simulink model "Byte_Demultiplexers"  (Simulink 8.1)
settings: Solver=ode45  StartTime=0.0  StopTime=10.0  RelTol=1e-3
libraries: Common_Library x32, commutil2 x22, Computer_Library x17
settings Model: Creator=uzivatel  LastModifiedBy=uzivatel
settings DataIOCC: SignalLoggingSaveFormat=Dataset
settings OptimizationCC: ExpressionDepthLimit=128
settings DebuggingCC: FcnCallInpInsideContextMsg=EnableAllAsError
settings GRTTargetCC: CombineOutputUpdateFcns=on  GRTInterface=off

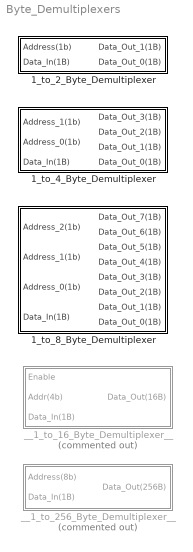
== system Byte_Demultiplexers ==
  1_to_2_Byte_Demultiplexer : Subsystem
  1_to_4_Byte_Demultiplexer : Subsystem
  1_to_8_Byte_Demultiplexer : Subsystem
  __1_to_16_Byte_Demultiplexer__ : Subsystem  Commented=on
  __1_to_256_Byte_Demultiplexer__ : Subsystem  Commented=on

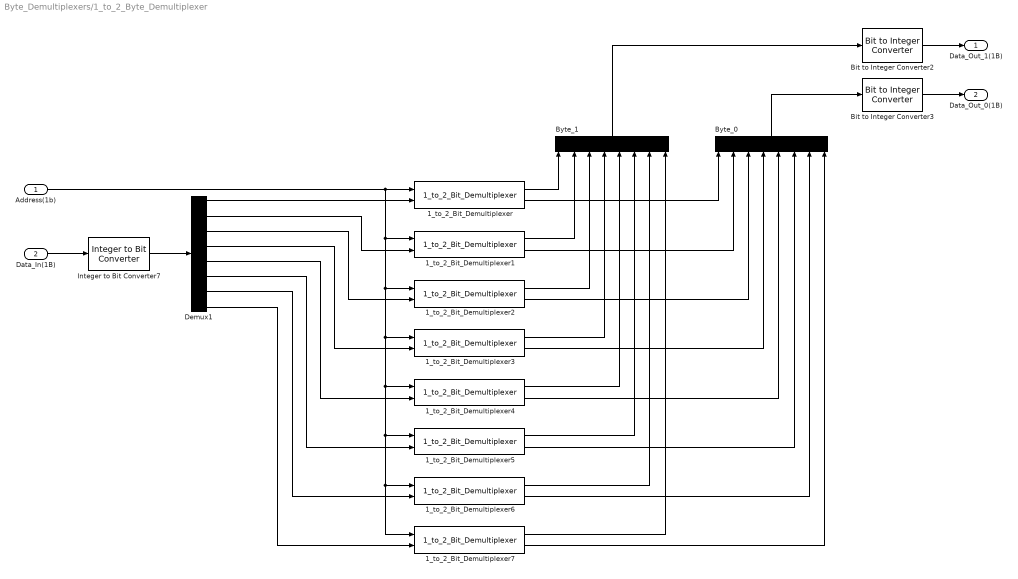
== system Byte_Demultiplexers/1_to_2_Byte_Demultiplexer ==
  Address(1b) : Inport
  Data_In(1B) : Inport  Port=2
  1_to_2_Bit_Demultiplexer{,1..7} (8 alike) : Common_Library/Demultiplexers/1_to_2_Bit_Demultiplexer
  Bit to Integer Converter2 : commutil2/Bit to Integer Converter  nbits=8  bitOrder=MSB first  signedOutputValues=Unsigned  outDtype=uint8  outDtypeSigned=Inherit via internal rule
  Bit to Integer Converter3 : commutil2/Bit to Integer Converter  nbits=8  bitOrder=MSB first  signedOutputValues=Unsigned  outDtype=uint8  outDtypeSigned=Inherit via internal rule
  Byte_0 : Mux  Inputs=8
  Byte_1 : Mux  Inputs=8
  Demux1 : Demux  Outputs=8
  Integer to Bit Converter7 : commutil2/Integer to Bit Converter  nbits=8  signedInputValues=Unsigned  bitOrder=MSB first  outDtype=boolean
  Data_Out_1(1B) : Outport
  Data_Out_0(1B) : Outport  Port=2
  wires:
  Demux1/4 -> 1_to_2_Bit_Demultiplexer3/2
  Demux1/5 -> 1_to_2_Bit_Demultiplexer4/2
  Demux1/6 -> 1_to_2_Bit_Demultiplexer5/2
  Demux1/7 -> 1_to_2_Bit_Demultiplexer6/2
  Demux1/8 -> 1_to_2_Bit_Demultiplexer7/2
  Demux1/3 -> 1_to_2_Bit_Demultiplexer2/2
  Demux1/2 -> 1_to_2_Bit_Demultiplexer1/2
  Demux1/1 -> 1_to_2_Bit_Demultiplexer/2
  Byte_1/1 -> Bit to Integer Converter2/1
  Byte_0/1 -> Bit to Integer Converter3/1
  1_to_2_Bit_Demultiplexer7/2 -> Byte_0/8
  1_to_2_Bit_Demultiplexer7/1 -> Byte_1/8
  1_to_2_Bit_Demultiplexer6/2 -> Byte_0/7
  1_to_2_Bit_Demultiplexer6/1 -> Byte_1/7
  1_to_2_Bit_Demultiplexer5/2 -> Byte_0/6
  1_to_2_Bit_Demultiplexer5/1 -> Byte_1/6
  1_to_2_Bit_Demultiplexer4/2 -> Byte_0/5
  1_to_2_Bit_Demultiplexer4/1 -> Byte_1/5
  1_to_2_Bit_Demultiplexer3/2 -> Byte_0/4
  1_to_2_Bit_Demultiplexer3/1 -> Byte_1/4
  1_to_2_Bit_Demultiplexer2/2 -> Byte_0/3
  1_to_2_Bit_Demultiplexer2/1 -> Byte_1/3
  1_to_2_Bit_Demultiplexer1/2 -> Byte_0/2
  1_to_2_Bit_Demultiplexer1/1 -> Byte_1/2
  1_to_2_Bit_Demultiplexer/2 -> Byte_0/1
  1_to_2_Bit_Demultiplexer/1 -> Byte_1/1
  Integer to Bit Converter7/1 -> Demux1/1
  Data_In(1B)/1 -> Integer to Bit Converter7/1
  Address(1b)/1 -> 1_to_2_Bit_Demultiplexer/1, 1_to_2_Bit_Demultiplexer7/1, 1_to_2_Bit_Demultiplexer6/1, 1_to_2_Bit_Demultiplexer5/1, 1_to_2_Bit_Demultiplexer4/1, 1_to_2_Bit_Demultiplexer3/1, 1_to_2_Bit_Demultiplexer2/1, 1_to_2_Bit_Demultiplexer1/1
  Bit to Integer Converter2/1 -> Data_Out_1(1B)/1
  Bit to Integer Converter3/1 -> Data_Out_0(1B)/1

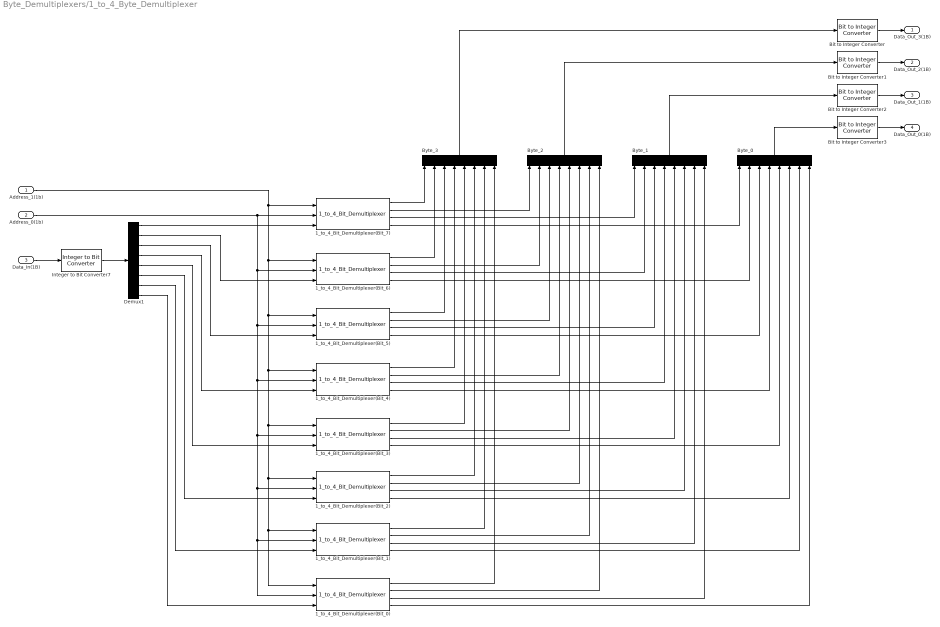
== system Byte_Demultiplexers/1_to_4_Byte_Demultiplexer ==
  Address_1(1b) : Inport
  Address_0(1b) : Inport  Port=2
  Data_In(1B) : Inport  Port=3
  1_to_4_Bit_Demultiplexer(Bit_0) : Common_Library/Demultiplexers/1_to_4_Bit_Demultiplexer
  1_to_4_Bit_Demultiplexer(Bit_1) : Common_Library/Demultiplexers/1_to_4_Bit_Demultiplexer
  1_to_4_Bit_Demultiplexer(Bit_2) : Common_Library/Demultiplexers/1_to_4_Bit_Demultiplexer
  1_to_4_Bit_Demultiplexer(Bit_3) : Common_Library/Demultiplexers/1_to_4_Bit_Demultiplexer
  1_to_4_Bit_Demultiplexer(Bit_4) : Common_Library/Demultiplexers/1_to_4_Bit_Demultiplexer
  1_to_4_Bit_Demultiplexer(Bit_5) : Common_Library/Demultiplexers/1_to_4_Bit_Demultiplexer
  1_to_4_Bit_Demultiplexer(Bit_6) : Common_Library/Demultiplexers/1_to_4_Bit_Demultiplexer
  1_to_4_Bit_Demultiplexer(Bit_7) : Common_Library/Demultiplexers/1_to_4_Bit_Demultiplexer
  Bit to Integer Converter{,1..3} (4 alike) : commutil2/Bit to Integer Converter  nbits=8  bitOrder=MSB first  signedOutputValues=Unsigned  outDtype=uint8  outDtypeSigned=Inherit via internal rule
  Byte_{0..3} (4 alike) : Mux  Inputs=8
  Demux1 : Demux  Outputs=8
  Integer to Bit Converter7 : commutil2/Integer to Bit Converter  nbits=8  signedInputValues=Unsigned  bitOrder=MSB first  outDtype=boolean
  Data_Out_3(1B) : Outport
  Data_Out_2(1B) : Outport  Port=2
  Data_Out_1(1B) : Outport  Port=3
  Data_Out_0(1B) : Outport  Port=4
  wires:
  Bit to Integer Converter/1 -> Data_Out_3(1B)/1
  Demux1/4 -> 1_to_4_Bit_Demultiplexer(Bit_4)/3
  Demux1/5 -> 1_to_4_Bit_Demultiplexer(Bit_3)/3
  Demux1/6 -> 1_to_4_Bit_Demultiplexer(Bit_2)/3
  Demux1/7 -> 1_to_4_Bit_Demultiplexer(Bit_1)/3
  Demux1/8 -> 1_to_4_Bit_Demultiplexer(Bit_0)/3
  Demux1/3 -> 1_to_4_Bit_Demultiplexer(Bit_5)/3
  Demux1/2 -> 1_to_4_Bit_Demultiplexer(Bit_6)/3
  Demux1/1 -> 1_to_4_Bit_Demultiplexer(Bit_7)/3
  Byte_3/1 -> Bit to Integer Converter/1
  Byte_2/1 -> Bit to Integer Converter1/1
  Byte_1/1 -> Bit to Integer Converter2/1
  Byte_0/1 -> Bit to Integer Converter3/1
  1_to_4_Bit_Demultiplexer(Bit_0)/4 -> Byte_0/8
  1_to_4_Bit_Demultiplexer(Bit_0)/3 -> Byte_1/8
  1_to_4_Bit_Demultiplexer(Bit_0)/2 -> Byte_2/8
  1_to_4_Bit_Demultiplexer(Bit_0)/1 -> Byte_3/8
  1_to_4_Bit_Demultiplexer(Bit_1)/4 -> Byte_0/7
  1_to_4_Bit_Demultiplexer(Bit_1)/3 -> Byte_1/7
  1_to_4_Bit_Demultiplexer(Bit_1)/2 -> Byte_2/7
  1_to_4_Bit_Demultiplexer(Bit_1)/1 -> Byte_3/7
  1_to_4_Bit_Demultiplexer(Bit_2)/4 -> Byte_0/6
  1_to_4_Bit_Demultiplexer(Bit_2)/3 -> Byte_1/6
  1_to_4_Bit_Demultiplexer(Bit_2)/2 -> Byte_2/6
  1_to_4_Bit_Demultiplexer(Bit_2)/1 -> Byte_3/6
  1_to_4_Bit_Demultiplexer(Bit_3)/4 -> Byte_0/5
  1_to_4_Bit_Demultiplexer(Bit_3)/3 -> Byte_1/5
  1_to_4_Bit_Demultiplexer(Bit_3)/2 -> Byte_2/5
  1_to_4_Bit_Demultiplexer(Bit_3)/1 -> Byte_3/5
  1_to_4_Bit_Demultiplexer(Bit_4)/4 -> Byte_0/4
  1_to_4_Bit_Demultiplexer(Bit_4)/3 -> Byte_1/4
  1_to_4_Bit_Demultiplexer(Bit_4)/2 -> Byte_2/4
  1_to_4_Bit_Demultiplexer(Bit_4)/1 -> Byte_3/4
  1_to_4_Bit_Demultiplexer(Bit_5)/4 -> Byte_0/3
  1_to_4_Bit_Demultiplexer(Bit_5)/3 -> Byte_1/3
  1_to_4_Bit_Demultiplexer(Bit_5)/2 -> Byte_2/3
  1_to_4_Bit_Demultiplexer(Bit_5)/1 -> Byte_3/3
  1_to_4_Bit_Demultiplexer(Bit_6)/4 -> Byte_0/2
  1_to_4_Bit_Demultiplexer(Bit_6)/3 -> Byte_1/2
  1_to_4_Bit_Demultiplexer(Bit_6)/2 -> Byte_2/2
  1_to_4_Bit_Demultiplexer(Bit_6)/1 -> Byte_3/2
  1_to_4_Bit_Demultiplexer(Bit_7)/4 -> Byte_0/1
  1_to_4_Bit_Demultiplexer(Bit_7)/3 -> Byte_1/1
  1_to_4_Bit_Demultiplexer(Bit_7)/2 -> Byte_2/1
  1_to_4_Bit_Demultiplexer(Bit_7)/1 -> Byte_3/1
  Integer to Bit Converter7/1 -> Demux1/1
  Data_In(1B)/1 -> Integer to Bit Converter7/1
  Address_0(1b)/1 -> 1_to_4_Bit_Demultiplexer(Bit_7)/2, 1_to_4_Bit_Demultiplexer(Bit_3)/2, 1_to_4_Bit_Demultiplexer(Bit_2)/2, 1_to_4_Bit_Demultiplexer(Bit_1)/2, 1_to_4_Bit_Demultiplexer(Bit_0)/2, 1_to_4_Bit_Demultiplexer(Bit_4)/2, 1_to_4_Bit_Demultiplexer(Bit_5)/2, 1_to_4_Bit_Demultiplexer(Bit_6)/2
  Address_1(1b)/1 -> 1_to_4_Bit_Demultiplexer(Bit_7)/1, 1_to_4_Bit_Demultiplexer(Bit_0)/1, 1_to_4_Bit_Demultiplexer(Bit_1)/1, 1_to_4_Bit_Demultiplexer(Bit_2)/1, 1_to_4_Bit_Demultiplexer(Bit_3)/1, 1_to_4_Bit_Demultiplexer(Bit_4)/1, 1_to_4_Bit_Demultiplexer(Bit_5)/1, 1_to_4_Bit_Demultiplexer(Bit_6)/1
  Bit to Integer Converter1/1 -> Data_Out_2(1B)/1
  Bit to Integer Converter2/1 -> Data_Out_1(1B)/1
  Bit to Integer Converter3/1 -> Data_Out_0(1B)/1

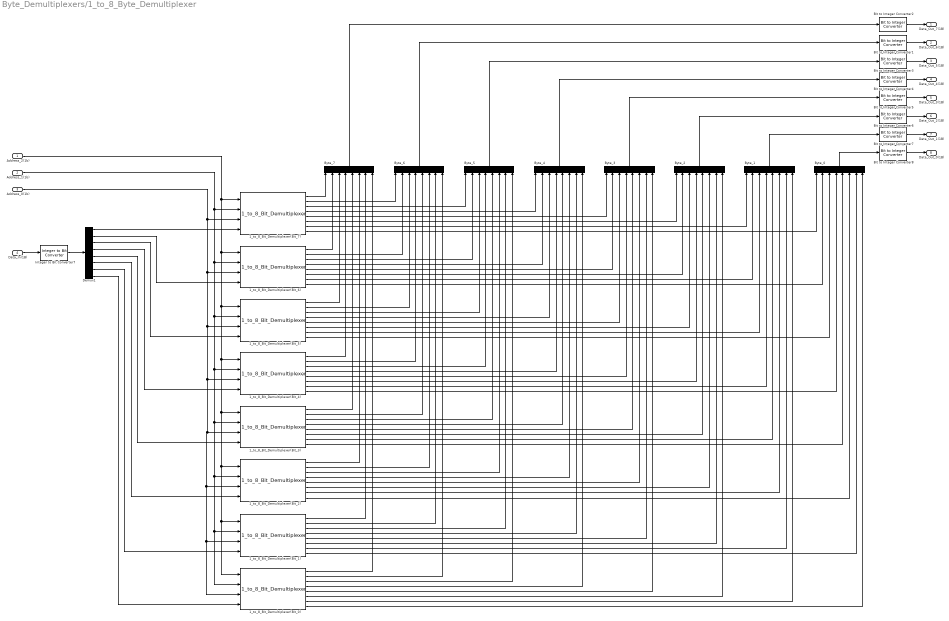
== system Byte_Demultiplexers/1_to_8_Byte_Demultiplexer ==
  Address_2(1b) : Inport
  Address_1(1b) : Inport  Port=2
  Address_0(1b) : Inport  Port=3
  Data_In(1B) : Inport  Port=4
  1_to_8_Bit_Demultiplexer(Bit_0) : Common_Library/Demultiplexers/1_to_8_Bit_Demultiplexer
  1_to_8_Bit_Demultiplexer(Bit_1) : Common_Library/Demultiplexers/1_to_8_Bit_Demultiplexer
  1_to_8_Bit_Demultiplexer(Bit_2) : Common_Library/Demultiplexers/1_to_8_Bit_Demultiplexer
  1_to_8_Bit_Demultiplexer(Bit_3) : Common_Library/Demultiplexers/1_to_8_Bit_Demultiplexer
  1_to_8_Bit_Demultiplexer(Bit_4) : Common_Library/Demultiplexers/1_to_8_Bit_Demultiplexer
  1_to_8_Bit_Demultiplexer(Bit_5) : Common_Library/Demultiplexers/1_to_8_Bit_Demultiplexer
  1_to_8_Bit_Demultiplexer(Bit_6) : Common_Library/Demultiplexers/1_to_8_Bit_Demultiplexer
  1_to_8_Bit_Demultiplexer(Bit_7) : Common_Library/Demultiplexers/1_to_8_Bit_Demultiplexer
  Bit to Integer Converter{1..8} (8 alike) : commutil2/Bit to Integer Converter  nbits=8  bitOrder=MSB first  signedOutputValues=Unsigned  outDtype=uint8  outDtypeSigned=Inherit via internal rule
  Byte_{0..7} (8 alike) : Mux  Inputs=8
  Demux1 : Demux  Outputs=8
  Integer to Bit Converter7 : commutil2/Integer to Bit Converter  nbits=8  signedInputValues=Unsigned  bitOrder=MSB first  outDtype=boolean
  Data_Out_7(1B) : Outport
  Data_Out_6(1B) : Outport  Port=2
  Data_Out_5(1B) : Outport  Port=3
  Data_Out_4(1B) : Outport  Port=4
  Data_Out_3(1B) : Outport  Port=5
  Data_Out_2(1B) : Outport  Port=6
  Data_Out_1(1B) : Outport  Port=7
  Data_Out_0(1B) : Outport  Port=8
  wires:
  Demux1/4 -> 1_to_8_Bit_Demultiplexer(Bit_4)/4
  Demux1/5 -> 1_to_8_Bit_Demultiplexer(Bit_3)/4
  Demux1/6 -> 1_to_8_Bit_Demultiplexer(Bit_2)/4
  Demux1/7 -> 1_to_8_Bit_Demultiplexer(Bit_1)/4
  Demux1/8 -> 1_to_8_Bit_Demultiplexer(Bit_0)/4
  Demux1/3 -> 1_to_8_Bit_Demultiplexer(Bit_5)/4
  Demux1/2 -> 1_to_8_Bit_Demultiplexer(Bit_6)/4
  Demux1/1 -> 1_to_8_Bit_Demultiplexer(Bit_7)/4
  Byte_7/1 -> Bit to Integer Converter2/1
  Byte_6/1 -> Bit to Integer Converter1/1
  Byte_5/1 -> Bit to Integer Converter3/1
  Byte_4/1 -> Bit to Integer Converter4/1
  Byte_3/1 -> Bit to Integer Converter5/1
  Byte_2/1 -> Bit to Integer Converter6/1
  Byte_1/1 -> Bit to Integer Converter7/1
  Byte_0/1 -> Bit to Integer Converter8/1
  1_to_8_Bit_Demultiplexer(Bit_0)/8 -> Byte_0/8
  1_to_8_Bit_Demultiplexer(Bit_0)/7 -> Byte_1/8
  1_to_8_Bit_Demultiplexer(Bit_0)/6 -> Byte_2/8
  1_to_8_Bit_Demultiplexer(Bit_0)/5 -> Byte_3/8
  1_to_8_Bit_Demultiplexer(Bit_0)/4 -> Byte_4/8
  1_to_8_Bit_Demultiplexer(Bit_0)/3 -> Byte_5/8
  1_to_8_Bit_Demultiplexer(Bit_0)/2 -> Byte_6/8
  1_to_8_Bit_Demultiplexer(Bit_0)/1 -> Byte_7/8
  1_to_8_Bit_Demultiplexer(Bit_1)/8 -> Byte_0/7
  1_to_8_Bit_Demultiplexer(Bit_1)/7 -> Byte_1/7
  1_to_8_Bit_Demultiplexer(Bit_1)/6 -> Byte_2/7
  1_to_8_Bit_Demultiplexer(Bit_1)/5 -> Byte_3/7
  1_to_8_Bit_Demultiplexer(Bit_1)/4 -> Byte_4/7
  1_to_8_Bit_Demultiplexer(Bit_1)/3 -> Byte_5/7
  1_to_8_Bit_Demultiplexer(Bit_1)/2 -> Byte_6/7
  1_to_8_Bit_Demultiplexer(Bit_1)/1 -> Byte_7/7
  1_to_8_Bit_Demultiplexer(Bit_2)/8 -> Byte_0/6
  1_to_8_Bit_Demultiplexer(Bit_2)/7 -> Byte_1/6
  1_to_8_Bit_Demultiplexer(Bit_2)/6 -> Byte_2/6
  1_to_8_Bit_Demultiplexer(Bit_2)/5 -> Byte_3/6
  1_to_8_Bit_Demultiplexer(Bit_2)/4 -> Byte_4/6
  1_to_8_Bit_Demultiplexer(Bit_2)/3 -> Byte_5/6
  1_to_8_Bit_Demultiplexer(Bit_2)/2 -> Byte_6/6
  1_to_8_Bit_Demultiplexer(Bit_2)/1 -> Byte_7/6
  1_to_8_Bit_Demultiplexer(Bit_3)/8 -> Byte_0/5
  1_to_8_Bit_Demultiplexer(Bit_3)/7 -> Byte_1/5
  1_to_8_Bit_Demultiplexer(Bit_3)/6 -> Byte_2/5
  1_to_8_Bit_Demultiplexer(Bit_3)/5 -> Byte_3/5
  1_to_8_Bit_Demultiplexer(Bit_3)/4 -> Byte_4/5
  1_to_8_Bit_Demultiplexer(Bit_3)/3 -> Byte_5/5
  1_to_8_Bit_Demultiplexer(Bit_3)/2 -> Byte_6/5
  1_to_8_Bit_Demultiplexer(Bit_3)/1 -> Byte_7/5
  1_to_8_Bit_Demultiplexer(Bit_4)/8 -> Byte_0/4
  1_to_8_Bit_Demultiplexer(Bit_4)/7 -> Byte_1/4
  1_to_8_Bit_Demultiplexer(Bit_4)/6 -> Byte_2/4
  1_to_8_Bit_Demultiplexer(Bit_4)/5 -> Byte_3/4
  1_to_8_Bit_Demultiplexer(Bit_4)/4 -> Byte_4/4
  1_to_8_Bit_Demultiplexer(Bit_4)/3 -> Byte_5/4
  1_to_8_Bit_Demultiplexer(Bit_4)/2 -> Byte_6/4
  1_to_8_Bit_Demultiplexer(Bit_4)/1 -> Byte_7/4
  1_to_8_Bit_Demultiplexer(Bit_5)/8 -> Byte_0/3
  1_to_8_Bit_Demultiplexer(Bit_5)/7 -> Byte_1/3
  1_to_8_Bit_Demultiplexer(Bit_5)/6 -> Byte_2/3
  1_to_8_Bit_Demultiplexer(Bit_5)/5 -> Byte_3/3
  1_to_8_Bit_Demultiplexer(Bit_5)/4 -> Byte_4/3
  1_to_8_Bit_Demultiplexer(Bit_5)/3 -> Byte_5/3
  1_to_8_Bit_Demultiplexer(Bit_5)/2 -> Byte_6/3
  1_to_8_Bit_Demultiplexer(Bit_5)/1 -> Byte_7/3
  1_to_8_Bit_Demultiplexer(Bit_6)/8 -> Byte_0/2
  1_to_8_Bit_Demultiplexer(Bit_6)/7 -> Byte_1/2
  1_to_8_Bit_Demultiplexer(Bit_6)/6 -> Byte_2/2
  1_to_8_Bit_Demultiplexer(Bit_6)/5 -> Byte_3/2
  1_to_8_Bit_Demultiplexer(Bit_6)/4 -> Byte_4/2
  1_to_8_Bit_Demultiplexer(Bit_6)/3 -> Byte_5/2
  1_to_8_Bit_Demultiplexer(Bit_6)/2 -> Byte_6/2
  1_to_8_Bit_Demultiplexer(Bit_6)/1 -> Byte_7/2
  1_to_8_Bit_Demultiplexer(Bit_7)/8 -> Byte_0/1
  1_to_8_Bit_Demultiplexer(Bit_7)/7 -> Byte_1/1
  1_to_8_Bit_Demultiplexer(Bit_7)/6 -> Byte_2/1
  1_to_8_Bit_Demultiplexer(Bit_7)/5 -> Byte_3/1
  1_to_8_Bit_Demultiplexer(Bit_7)/4 -> Byte_4/1
  1_to_8_Bit_Demultiplexer(Bit_7)/3 -> Byte_5/1
  1_to_8_Bit_Demultiplexer(Bit_7)/2 -> Byte_6/1
  1_to_8_Bit_Demultiplexer(Bit_7)/1 -> Byte_7/1
  Integer to Bit Converter7/1 -> Demux1/1
  Data_In(1B)/1 -> Integer to Bit Converter7/1
  Address_0(1b)/1 -> 1_to_8_Bit_Demultiplexer(Bit_7)/3, 1_to_8_Bit_Demultiplexer(Bit_6)/3, 1_to_8_Bit_Demultiplexer(Bit_5)/3, 1_to_8_Bit_Demultiplexer(Bit_0)/3, 1_to_8_Bit_Demultiplexer(Bit_1)/3, 1_to_8_Bit_Demultiplexer(Bit_2)/3, 1_to_8_Bit_Demultiplexer(Bit_3)/3, 1_to_8_Bit_Demultiplexer(Bit_4)/3
  Address_1(1b)/1 -> 1_to_8_Bit_Demultiplexer(Bit_7)/2, 1_to_8_Bit_Demultiplexer(Bit_0)/2, 1_to_8_Bit_Demultiplexer(Bit_1)/2, 1_to_8_Bit_Demultiplexer(Bit_2)/2, 1_to_8_Bit_Demultiplexer(Bit_3)/2, 1_to_8_Bit_Demultiplexer(Bit_4)/2, 1_to_8_Bit_Demultiplexer(Bit_5)/2, 1_to_8_Bit_Demultiplexer(Bit_6)/2
  Address_2(1b)/1 -> 1_to_8_Bit_Demultiplexer(Bit_7)/1, 1_to_8_Bit_Demultiplexer(Bit_0)/1, 1_to_8_Bit_Demultiplexer(Bit_1)/1, 1_to_8_Bit_Demultiplexer(Bit_2)/1, 1_to_8_Bit_Demultiplexer(Bit_3)/1, 1_to_8_Bit_Demultiplexer(Bit_4)/1, 1_to_8_Bit_Demultiplexer(Bit_5)/1, 1_to_8_Bit_Demultiplexer(Bit_6)/1
  Bit to Integer Converter8/1 -> Data_Out_0(1B)/1
  Bit to Integer Converter7/1 -> Data_Out_1(1B)/1
  Bit to Integer Converter6/1 -> Data_Out_2(1B)/1
  Bit to Integer Converter5/1 -> Data_Out_3(1B)/1
  Bit to Integer Converter4/1 -> Data_Out_4(1B)/1
  Bit to Integer Converter3/1 -> Data_Out_5(1B)/1
  Bit to Integer Converter1/1 -> Data_Out_6(1B)/1
  Bit to Integer Converter2/1 -> Data_Out_7(1B)/1

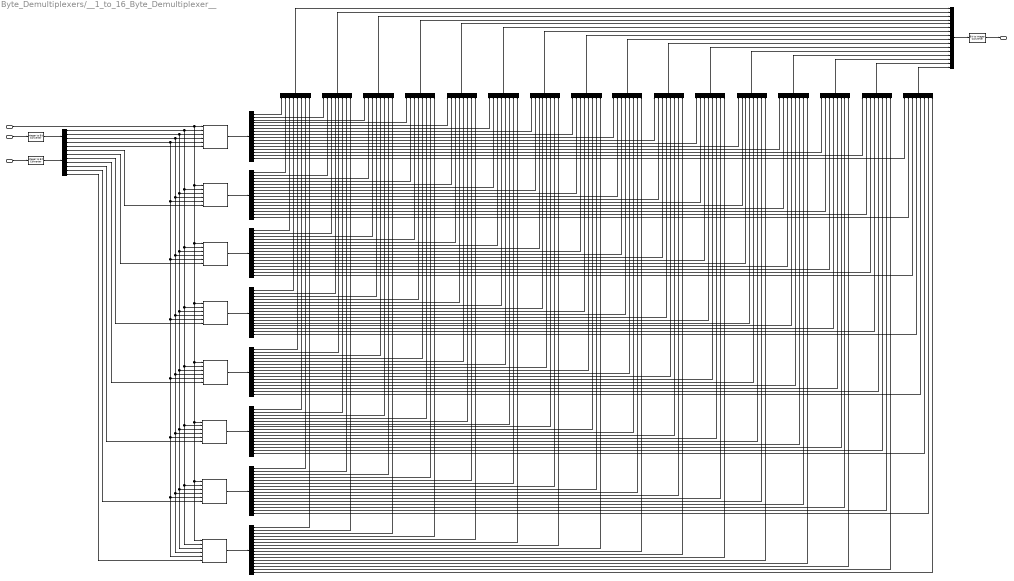
== system Byte_Demultiplexers/__1_to_16_Byte_Demultiplexer__ ==
  Enable : Inport
  Addr(4b) : Inport  Port=2
  Data_In(1B) : Inport  Port=3
  1_to_16_Bit_Demultiplexer(Bit_0) : Common_Library/Demultiplexers/1_to_16_Bit_Demultiplexer
  1_to_16_Bit_Demultiplexer(Bit_1) : Common_Library/Demultiplexers/1_to_16_Bit_Demultiplexer
  1_to_16_Bit_Demultiplexer(Bit_2) : Common_Library/Demultiplexers/1_to_16_Bit_Demultiplexer
  1_to_16_Bit_Demultiplexer(Bit_3) : Common_Library/Demultiplexers/1_to_16_Bit_Demultiplexer
  1_to_16_Bit_Demultiplexer(Bit_4) : Common_Library/Demultiplexers/1_to_16_Bit_Demultiplexer
  1_to_16_Bit_Demultiplexer(Bit_5) : Common_Library/Demultiplexers/1_to_16_Bit_Demultiplexer
  1_to_16_Bit_Demultiplexer(Bit_6) : Common_Library/Demultiplexers/1_to_16_Bit_Demultiplexer
  1_to_16_Bit_Demultiplexer(Bit_7) : Common_Library/Demultiplexers/1_to_16_Bit_Demultiplexer
  Bit to Integer Converter : commutil2/Bit to Integer Converter  nbits=8  bitOrder=MSB first  signedOutputValues=Unsigned  outDtype=uint8  outDtypeSigned=Inherit via internal rule
  Bit_{0..7} (8 alike) : Demux  Outputs=16
  Byte_{0..15} (16 alike) : Mux  Inputs=8
  Demux1 : Demux  Outputs=8
  Demux17 : Demux
  Integer to Bit Converter5 : commutil2/Integer to Bit Converter  nbits=4  signedInputValues=Unsigned  bitOrder=MSB first  outDtype=int8
  Integer to Bit Converter7 : commutil2/Integer to Bit Converter  nbits=8  signedInputValues=Unsigned  bitOrder=MSB first  outDtype=boolean
  Mux1 : Mux  Inputs=16
  Data_Out(16B) : Outport
  wires:
  Bit to Integer Converter/1 -> Data_Out(16B)/1
  Mux1/1 -> Bit to Integer Converter/1
  Addr(4b)/1 -> Integer to Bit Converter5/1
  Integer to Bit Converter5/1 -> Demux17/1
  Enable/1 -> 1_to_16_Bit_Demultiplexer(Bit_0)/1, 1_to_16_Bit_Demultiplexer(Bit_1)/1, 1_to_16_Bit_Demultiplexer(Bit_2)/1, 1_to_16_Bit_Demultiplexer(Bit_3)/1, 1_to_16_Bit_Demultiplexer(Bit_4)/1, 1_to_16_Bit_Demultiplexer(Bit_5)/1, 1_to_16_Bit_Demultiplexer(Bit_6)/1, 1_to_16_Bit_Demultiplexer(Bit_7)/1
  Demux1/4 -> 1_to_16_Bit_Demultiplexer(Bit_4)/6
  Demux1/5 -> 1_to_16_Bit_Demultiplexer(Bit_3)/6
  Demux1/6 -> 1_to_16_Bit_Demultiplexer(Bit_2)/6
  Demux1/7 -> 1_to_16_Bit_Demultiplexer(Bit_1)/6
  Demux1/8 -> 1_to_16_Bit_Demultiplexer(Bit_0)/6
  Demux1/3 -> 1_to_16_Bit_Demultiplexer(Bit_5)/6
  Demux1/2 -> 1_to_16_Bit_Demultiplexer(Bit_6)/6
  Demux1/1 -> 1_to_16_Bit_Demultiplexer(Bit_7)/6
  Byte_15/1 -> Mux1/1
  Byte_14/1 -> Mux1/2
  Byte_13/1 -> Mux1/3
  Byte_12/1 -> Mux1/4
  Byte_11/1 -> Mux1/5
  Byte_10/1 -> Mux1/6
  Byte_9/1 -> Mux1/7
  Byte_8/1 -> Mux1/8
  Byte_7/1 -> Mux1/9
  Byte_6/1 -> Mux1/10
  Byte_5/1 -> Mux1/11
  Byte_4/1 -> Mux1/12
  Byte_3/1 -> Mux1/13
  Byte_2/1 -> Mux1/14
  Byte_1/1 -> Mux1/15
  Byte_0/1 -> Mux1/16
  Bit_0/16 -> Byte_0/8
  Bit_0/15 -> Byte_1/8
  Bit_0/14 -> Byte_2/8
  Bit_0/13 -> Byte_3/8
  Bit_0/12 -> Byte_4/8
  Bit_0/11 -> Byte_5/8
  Bit_0/10 -> Byte_6/8
  Bit_0/9 -> Byte_7/8
  Bit_0/8 -> Byte_8/8
  Bit_0/7 -> Byte_9/8
  Bit_0/6 -> Byte_10/8
  Bit_0/5 -> Byte_11/8
  Bit_0/4 -> Byte_12/8
  Bit_0/3 -> Byte_13/8
  Bit_0/2 -> Byte_14/8
  Bit_0/1 -> Byte_15/8
  Bit_1/16 -> Byte_0/7
  Bit_1/15 -> Byte_1/7
  Bit_1/14 -> Byte_2/7
  Bit_1/13 -> Byte_3/7
  Bit_1/12 -> Byte_4/7
  Bit_1/11 -> Byte_5/7
  Bit_1/10 -> Byte_6/7
  Bit_1/9 -> Byte_7/7
  Bit_1/8 -> Byte_8/7
  Bit_1/7 -> Byte_9/7
  Bit_1/6 -> Byte_10/7
  Bit_1/5 -> Byte_11/7
  Bit_1/4 -> Byte_12/7
  Bit_1/3 -> Byte_13/7
  Bit_1/2 -> Byte_14/7
  Bit_1/1 -> Byte_15/7
  Bit_2/16 -> Byte_0/6
  Bit_2/15 -> Byte_1/6
  Bit_2/14 -> Byte_2/6
  Bit_2/13 -> Byte_3/6
  Bit_2/12 -> Byte_4/6
  Bit_2/11 -> Byte_5/6
  Bit_2/10 -> Byte_6/6
  Bit_2/9 -> Byte_7/6
  Bit_2/8 -> Byte_8/6
  Bit_2/7 -> Byte_9/6
  Bit_2/6 -> Byte_10/6
  Bit_2/5 -> Byte_11/6
  Bit_2/4 -> Byte_12/6
  Bit_2/3 -> Byte_13/6
  Bit_2/2 -> Byte_14/6
  Bit_2/1 -> Byte_15/6
  Bit_3/16 -> Byte_0/5
  Bit_3/15 -> Byte_1/5
  Bit_3/14 -> Byte_2/5
  Bit_3/13 -> Byte_3/5
  Bit_3/12 -> Byte_4/5
  Bit_3/11 -> Byte_5/5
  Bit_3/10 -> Byte_6/5
  Bit_3/9 -> Byte_7/5
  Bit_3/8 -> Byte_8/5
  Bit_3/7 -> Byte_9/5
  Bit_3/6 -> Byte_10/5
  Bit_3/5 -> Byte_11/5
  Bit_3/4 -> Byte_12/5
  Bit_3/3 -> Byte_13/5
  Bit_3/2 -> Byte_14/5
  Bit_3/1 -> Byte_15/5
  Bit_4/16 -> Byte_0/4
  Bit_4/15 -> Byte_1/4
  Bit_4/14 -> Byte_2/4
  Bit_4/13 -> Byte_3/4
  Bit_4/12 -> Byte_4/4
  Bit_4/11 -> Byte_5/4
  Bit_4/10 -> Byte_6/4
  Bit_4/9 -> Byte_7/4
  Bit_4/8 -> Byte_8/4
  Bit_4/7 -> Byte_9/4
  Bit_4/6 -> Byte_10/4
  Bit_4/5 -> Byte_11/4
  Bit_4/4 -> Byte_12/4
  Bit_4/3 -> Byte_13/4
  Bit_4/2 -> Byte_14/4
  Bit_4/1 -> Byte_15/4
  Bit_5/16 -> Byte_0/3
  Bit_5/15 -> Byte_1/3
  Bit_5/14 -> Byte_2/3
  Bit_5/13 -> Byte_3/3
  Bit_5/12 -> Byte_4/3
  Bit_5/11 -> Byte_5/3
  Bit_5/10 -> Byte_6/3
  Bit_5/9 -> Byte_7/3
  Bit_5/8 -> Byte_8/3
  Bit_5/7 -> Byte_9/3
  Bit_5/6 -> Byte_10/3
  Bit_5/5 -> Byte_11/3
  Bit_5/4 -> Byte_12/3
  Bit_5/3 -> Byte_13/3
  Bit_5/2 -> Byte_14/3
  Bit_5/1 -> Byte_15/3
  Bit_6/16 -> Byte_0/2
  Bit_6/15 -> Byte_1/2
  Bit_6/14 -> Byte_2/2
  Bit_6/13 -> Byte_3/2
  Bit_6/12 -> Byte_4/2
  Bit_6/11 -> Byte_5/2
  Bit_6/10 -> Byte_6/2
  Bit_6/9 -> Byte_7/2
  Bit_6/8 -> Byte_8/2
  Bit_6/7 -> Byte_9/2
  Bit_6/6 -> Byte_10/2
  Bit_6/5 -> Byte_11/2
  Bit_6/4 -> Byte_12/2
  Bit_6/3 -> Byte_13/2
  Bit_6/2 -> Byte_14/2
  Bit_6/1 -> Byte_15/2
  Bit_7/16 -> Byte_0/1
  Bit_7/15 -> Byte_1/1
  Bit_7/14 -> Byte_2/1
  Bit_7/13 -> Byte_3/1
  Bit_7/12 -> Byte_4/1
  Bit_7/11 -> Byte_5/1
  Bit_7/10 -> Byte_6/1
  Bit_7/9 -> Byte_7/1
  Bit_7/8 -> Byte_8/1
  Bit_7/7 -> Byte_9/1
  Bit_7/6 -> Byte_10/1
  Bit_7/5 -> Byte_11/1
  Bit_7/4 -> Byte_12/1
  Bit_7/3 -> Byte_13/1
  Bit_7/2 -> Byte_14/1
  Bit_7/1 -> Byte_15/1
  1_to_16_Bit_Demultiplexer(Bit_0)/1 -> Bit_0/1
  1_to_16_Bit_Demultiplexer(Bit_1)/1 -> Bit_1/1
  1_to_16_Bit_Demultiplexer(Bit_2)/1 -> Bit_2/1
  1_to_16_Bit_Demultiplexer(Bit_3)/1 -> Bit_3/1
  1_to_16_Bit_Demultiplexer(Bit_4)/1 -> Bit_4/1
  1_to_16_Bit_Demultiplexer(Bit_5)/1 -> Bit_5/1
  1_to_16_Bit_Demultiplexer(Bit_6)/1 -> Bit_6/1
  1_to_16_Bit_Demultiplexer(Bit_7)/1 -> Bit_7/1
  Integer to Bit Converter7/1 -> Demux1/1
  Data_In(1B)/1 -> Integer to Bit Converter7/1
  Demux17/4 -> 1_to_16_Bit_Demultiplexer(Bit_7)/5, 1_to_16_Bit_Demultiplexer(Bit_0)/5, 1_to_16_Bit_Demultiplexer(Bit_1)/5, 1_to_16_Bit_Demultiplexer(Bit_2)/5, 1_to_16_Bit_Demultiplexer(Bit_3)/5, 1_to_16_Bit_Demultiplexer(Bit_4)/5, 1_to_16_Bit_Demultiplexer(Bit_5)/5, 1_to_16_Bit_Demultiplexer(Bit_6)/5
  Demux17/3 -> 1_to_16_Bit_Demultiplexer(Bit_7)/4, 1_to_16_Bit_Demultiplexer(Bit_0)/4, 1_to_16_Bit_Demultiplexer(Bit_1)/4, 1_to_16_Bit_Demultiplexer(Bit_2)/4, 1_to_16_Bit_Demultiplexer(Bit_3)/4, 1_to_16_Bit_Demultiplexer(Bit_4)/4, 1_to_16_Bit_Demultiplexer(Bit_5)/4, 1_to_16_Bit_Demultiplexer(Bit_6)/4
  Demux17/2 -> 1_to_16_Bit_Demultiplexer(Bit_7)/3, 1_to_16_Bit_Demultiplexer(Bit_1)/3, 1_to_16_Bit_Demultiplexer(Bit_0)/3, 1_to_16_Bit_Demultiplexer(Bit_2)/3, 1_to_16_Bit_Demultiplexer(Bit_3)/3, 1_to_16_Bit_Demultiplexer(Bit_4)/3, 1_to_16_Bit_Demultiplexer(Bit_5)/3, 1_to_16_Bit_Demultiplexer(Bit_6)/3
  Demux17/1 -> 1_to_16_Bit_Demultiplexer(Bit_7)/2, 1_to_16_Bit_Demultiplexer(Bit_0)/2, 1_to_16_Bit_Demultiplexer(Bit_1)/2, 1_to_16_Bit_Demultiplexer(Bit_2)/2, 1_to_16_Bit_Demultiplexer(Bit_3)/2, 1_to_16_Bit_Demultiplexer(Bit_4)/2, 1_to_16_Bit_Demultiplexer(Bit_5)/2, 1_to_16_Bit_Demultiplexer(Bit_6)/2

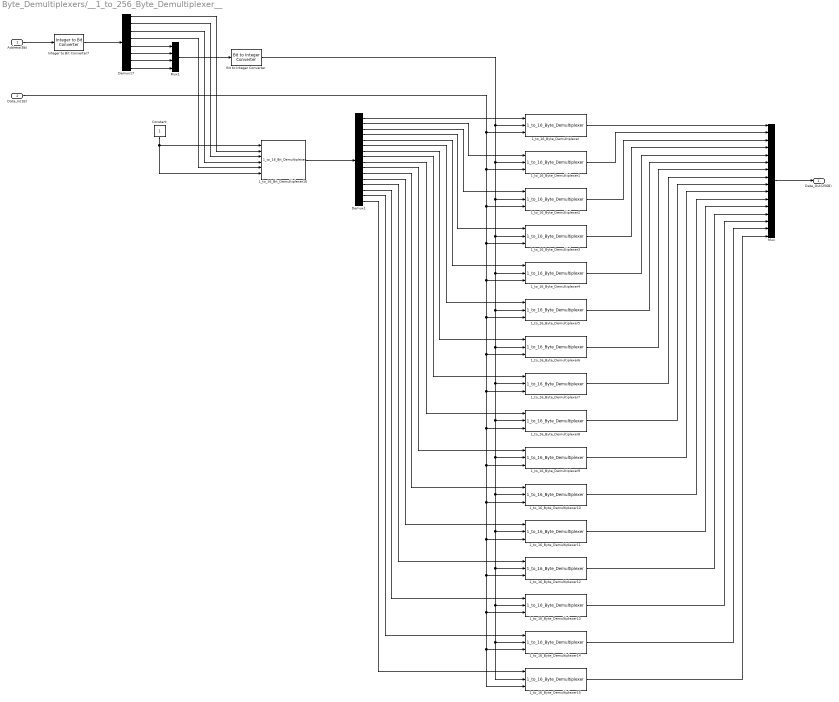
== system Byte_Demultiplexers/__1_to_256_Byte_Demultiplexer__ ==
  Address(8b) : Inport
  Data_In(1B) : Inport  Port=2
  1_to_16_Bit_Demultiplexer16 : Computer_Library/Demultiplexers/1_to_16_Bit_Demultiplexer
  1_to_16_Byte_Demultiplexer{,1..15} (16 alike) : Computer_Library/Demultiplexers/1_to_16_Byte_Demultiplexer
  Bit to Integer Converter : commutil2/Bit to Integer Converter  nbits=4  bitOrder=MSB first  signedOutputValues=Unsigned  outDtype=uint8  outDtypeSigned=Inherit via internal rule
  Constant : Constant
  Demux1 : Demux  Outputs=16
  Demux17 : Demux  Outputs=8
  Integer to Bit Converter7 : commutil2/Integer to Bit Converter  nbits=8  signedInputValues=Unsigned  bitOrder=MSB first  outDtype=boolean
  Mux : Mux  Inputs=16
  Mux1 : Mux
  Data_Out(256B) : Outport  OutDataTypeStr=uint8
  wires:
  Mux1/1 -> Bit to Integer Converter/1
  Address(8b)/1 -> Integer to Bit Converter7/1
  Integer to Bit Converter7/1 -> Demux17/1
  Bit to Integer Converter/1 -> 1_to_16_Byte_Demultiplexer2/2, 1_to_16_Byte_Demultiplexer3/2, 1_to_16_Byte_Demultiplexer4/2, 1_to_16_Byte_Demultiplexer15/2, 1_to_16_Byte_Demultiplexer14/2, 1_to_16_Byte_Demultiplexer13/2, 1_to_16_Byte_Demultiplexer12/2, 1_to_16_Byte_Demultiplexer11/2, 1_to_16_Byte_Demultiplexer10/2, 1_to_16_Byte_Demultiplexer9/2, 1_to_16_Byte_Demultiplexer8/2, 1_to_16_Byte_Demultiplexer7/2, 1_to_16_Byte_Demultiplexer6/2, 1_to_16_Byte_Demultiplexer5/2, 1_to_16_Byte_Demultiplexer1/2, 1_to_16_Byte_Demultiplexer/2
  Demux17/8 -> Mux1/4
  Demux17/7 -> Mux1/3
  Demux17/6 -> Mux1/2
  Demux17/5 -> Mux1/1
  Demux17/3 -> 1_to_16_Bit_Demultiplexer16/4
  Demux17/4 -> 1_to_16_Bit_Demultiplexer16/5
  Demux17/2 -> 1_to_16_Bit_Demultiplexer16/3
  Demux17/1 -> 1_to_16_Bit_Demultiplexer16/2
  Mux/1 -> Data_Out(256B)/1
  Constant/1 -> 1_to_16_Bit_Demultiplexer16/6, 1_to_16_Bit_Demultiplexer16/1
  Demux1/16 -> 1_to_16_Byte_Demultiplexer15/1
  Demux1/15 -> 1_to_16_Byte_Demultiplexer14/1
  Demux1/14 -> 1_to_16_Byte_Demultiplexer13/1
  Demux1/13 -> 1_to_16_Byte_Demultiplexer12/1
  Demux1/12 -> 1_to_16_Byte_Demultiplexer11/1
  Demux1/11 -> 1_to_16_Byte_Demultiplexer10/1
  Demux1/10 -> 1_to_16_Byte_Demultiplexer9/1
  Demux1/9 -> 1_to_16_Byte_Demultiplexer8/1
  Demux1/8 -> 1_to_16_Byte_Demultiplexer7/1
  Demux1/7 -> 1_to_16_Byte_Demultiplexer6/1
  Demux1/6 -> 1_to_16_Byte_Demultiplexer5/1
  Demux1/5 -> 1_to_16_Byte_Demultiplexer4/1
  Demux1/4 -> 1_to_16_Byte_Demultiplexer3/1
  Demux1/3 -> 1_to_16_Byte_Demultiplexer2/1
  Demux1/2 -> 1_to_16_Byte_Demultiplexer1/1
  Demux1/1 -> 1_to_16_Byte_Demultiplexer/1
  1_to_16_Bit_Demultiplexer16/1 -> Demux1/1
  Data_In(1B)/1 -> 1_to_16_Byte_Demultiplexer/3, 1_to_16_Byte_Demultiplexer1/3, 1_to_16_Byte_Demultiplexer2/3, 1_to_16_Byte_Demultiplexer3/3, 1_to_16_Byte_Demultiplexer4/3, 1_to_16_Byte_Demultiplexer5/3, 1_to_16_Byte_Demultiplexer6/3, 1_to_16_Byte_Demultiplexer7/3, 1_to_16_Byte_Demultiplexer8/3, 1_to_16_Byte_Demultiplexer9/3, 1_to_16_Byte_Demultiplexer10/3, 1_to_16_Byte_Demultiplexer11/3, 1_to_16_Byte_Demultiplexer12/3, 1_to_16_Byte_Demultiplexer13/3, 1_to_16_Byte_Demultiplexer14/3, 1_to_16_Byte_Demultiplexer15/3
  1_to_16_Byte_Demultiplexer/1 -> Mux/1
  1_to_16_Byte_Demultiplexer1/1 -> Mux/2
  1_to_16_Byte_Demultiplexer2/1 -> Mux/3
  1_to_16_Byte_Demultiplexer3/1 -> Mux/4
  1_to_16_Byte_Demultiplexer15/1 -> Mux/16
  1_to_16_Byte_Demultiplexer14/1 -> Mux/15
  1_to_16_Byte_Demultiplexer13/1 -> Mux/14
  1_to_16_Byte_Demultiplexer12/1 -> Mux/13
  1_to_16_Byte_Demultiplexer11/1 -> Mux/12
  1_to_16_Byte_Demultiplexer10/1 -> Mux/11
  1_to_16_Byte_Demultiplexer9/1 -> Mux/10
  1_to_16_Byte_Demultiplexer8/1 -> Mux/9
  1_to_16_Byte_Demultiplexer7/1 -> Mux/8
  1_to_16_Byte_Demultiplexer6/1 -> Mux/7
  1_to_16_Byte_Demultiplexer5/1 -> Mux/6
  1_to_16_Byte_Demultiplexer4/1 -> Mux/5
